simulink model "different_inverter_controls_BPS"  (R2024b)
settings: Solver=ode4  StartTime=0.0  StopTime=5  FixedStep=Ts  RelTol=1e-3
InitFcn:
  | %mode_of_operation=1;
  | %BESS_control_mode=1;
  | %Gen_Q_Control =1;
  | 
  | %Exciter_init;
  | 
  | %Exciter_init
  | Xq=0.474;
  | %%====================================================
  | % ST6C Exciter Parameters
  | 
  | KPA=30;
  | KIA=59.91;
  | KFF=1;
  | KM=1;
  | KLR=22.47;
  | KCL=1.04;
  | VAMAX=7.05;
  | VAMIN=-6.11;
  | VRMAX=7.05;
  | VRMIN=-6.11;
  | ILR=5.02;
  | KG=1;
  | TG=0.024;
  | TA=0.01;
  | VBMAX=999;
  | VMMAX=7.05;
  | VMMIN=-6.11;
  | KI=0;
  | Kp=1;
  | Kc=0;
  | Vt0=0;
  | VAAMAX=VAMAX;
  | %%========================================================
  | % UEL2C parameters
  | 
  | TUQ=.005;
  | TUP=0.050;
  | TUV=0.2;
  | TQREF=0;
  | Tadj=0;
  | K1=0;
  | K2=2;
  | VBIAS=1;
  | KFB=0;
  | TUL=0;
  | VUImax=1;
  | VUImin=-1;
  | VUELmax1=1;
  | VUELmax2=1;
  | VUELmin1=-1;
  | VUELmin2=-1;
  | KUF=0;
  | KUL=0.24;
  | KUI=0.001;
  | TU1=0;TU2=0;TU3=0;TU4=0;
  | KFIX=1;
  | VF=0;
  | VFB=0;
  | %%===========================================================
  | ... (+60 lines)
values from neighbouring files (symbols this model uses):
  inv1 = struct    [multiInverterParams.m]
  kp_sync = KQ_p/10    (= 0.04)    [multiInverterParams.m]
  Vdc = 1000    [multiInverterParams.m]
  Vpp = 480    [multiInverterParams.m]
undefined symbols (not defined in the file or in its folder): D1, Delta, DiscIntNeverNeededParam, Ion, Lithium, sigbuilder_block, sps
libraries: slpidlib x34, spsThreePhaseVIMeasurementLib x31, spsThreePhaseSeriesRLCBranchLib x23, spsabctodq0Lib x22, spsPower3phInstantaneousLib x22, spsThreePhaseTransformerTwoWindingsLib x16, spsSeriesRLCBranchLib x16, spsThreePhaseSeriesRLCLoadLib x14, simulink x12, spsPLL3phLib x11, spsGroundLib x9, powerlib_extras x8
(part 7 of 9)

== system different_inverter_controls_BPS/GFM-VSG-100MW/IBR-GFM VSG/Inverter/Power Controller/P,Q Control  ==
  PQref : Inport
  m : Inport  Port=2
  V_inv_mag : Inport  Port=3
  Constant2 : Constant  Value=0  SampleTime=Ts_Control
  Demux : Demux  Outputs=2
  Demux1 : Demux  Outputs=2
  Gain1 : Gain  Gain=77*10
  Integrator : Subsystem
  Reactive Controller : slpidlib/PID Controller  Controller=PI  Form=Parallel  TimeDomain=Discrete-time  UseExternalTs=off  SampleTime=Ts_Control  IntegratorMethod=Forward Euler  FilterMethod=Forward Euler  ControllerParametersSource=internal  P=-.001  I=0  UseKiTs=off  D=0  UseExternalDerivativeSource=off  N=100  UseFilter=on  TunerSelectOption=Transfer Function Based (PID Tuner App)  InitialConditionSource=internal  InitialConditionForIntegrator=0  InitialConditionForFilter=0  DifferentiatorICPrevScaledInput=0  ExternalReset=none  TrackingMode=off  Kt=1  LimitOutput=on  SatLimitsSource=internal  UpperSaturationLimit=1.5  LowerSaturationLimit=-1.5  LinearizeAsGain=off  AntiWindupMode=back-calculation  Kb=1  LimitIntegrator=off  UpperIntegratorSaturationLimit=inf  LowerIntegratorSaturationLimit=-inf  POutMin=[]  POutMax=[]  IOutMin=[]  IOutMax=[]  DOutMin=[]  DOutMax=[]  NOutMin=[]  NOutMax=[]  SumOutMin=[]  SumOutMax=[]  SaturationOutMin=[]  SaturationOutMax=[]  PParamMin=[]  PParamMax=[]  IParamMin=[]  IParamMax=[]  DParamMin=[]  DParamMax=[]  NParamMin=[]  NParamMax=[]  KbParamMin=[]  KbParamMax=[]  KtParamMin=[]  KtParamMax=[]  KbOutMin=[]  KbOutMax=[]  KtOutMin=[]  KtOutMax=[]  IntegratorOutMin=[]  IntegratorOutMax=[]  FilterOutMin=[]  FilterOutMax=[]  SumI1OutMin=[]  SumI1OutMax=[]  SumI2OutMin=[]  SumI2OutMax=[]  SumI3OutMin=[]  SumI3OutMax=[]  SumI4OutMin=[]  SumI4OutMax=[]  SumDOutMin=[]  SumDOutMax=[]  DifferentiatorOutMin=[]  DifferentiatorOutMax=[]  FilterDiffOutCoefMin=[]  FilterDiffOutCoefMax=[]  ReciprocalOutMin=[]  ReciprocalOutMax=[]  SumDenOutMin=[]  SumDenOutMax=[]  SumNumOutMin=[]  SumNumOutMax=[]  DivideOutMin=[]  DivideOutMax=[]  UdiffTsProdOutMin=[]  UdiffTsProdOutMax=[]  NTsProdOutMin=[]  NTsProdOutMax=[]  UintegralTsProdOutMin=[]  UintegralTsProdOutMax=[]  UngainTsProdOutMin=[]  UngainTsProdOutMax=[]  ClampingZeroOutDataTypeStr=Inherit: Inherit via back propagation  ClampingZeroOutMin=[]  ClampingZeroOutMax=[]  FilterDenConstantOutDataTypeStr=Inherit: Inherit via back propagation  FilterDenConstantOutMin=[]  FilterDenConstantOutMax=[]  PCopyOutDataTypeStr=Inherit: Inherit via back propagation  PCopyOutMin=[]  PCopyOutMax=[]  NCopyOutDataTypeStr=Inherit: Inherit via back propagation  NCopyOutMin=[]  NCopyOutMax=[]  IntegratorContinuousStateAttributes=''  IntegratorStateMustResolveToSignalObject=off  IntegratorRTWStateStorageClass=Auto  FilterContinuousStateAttributes=''  FilterStateMustResolveToSignalObject=off  FilterRTWStateStorageClass=Auto  ParallelPVariant=InternalParameters  IdealPVariant=Disabled  IVariant=InternalParameters  DVariant=Disabled  IntegratorVariant=Discrete  SatVariant=Enabled  AWVariant=BackCalculation  PCopyVariant=Disabled  TRVariant=Disabled  FdbkBlocksVariant=Forward  IdealPFdbkVariant=Disabled  SatFdbkVariant=Disabled  DerivativeFilterVariant=Disabled  NVariant=Disabled  NCopyVariant=Disabled_SignalSpec  FilterICVariant=Disabled  IntegratorICVariant=InternalICs  ExternalResetVariant=Disabled  TRSumVariant=Passthrough  SumFdbkVariant=Disabled  SumVariant=Sum_PI  TsampFilterVariant=InternalTs  TsampNgainVariant=Passthrough  TsampIntegralVariant=Disabled_SignalSpec  ExternalSaturationOutDataTypeStr=Inherit: Same as second input  DerivativeSourceVariant=Disabled  PreIntVariant=InternalPreInt
  Scope{1,3,6..9} (6 alike) : Scope
  Scope10 : Scope  NumInputPorts=2
  Scope2 : Scope  NumInputPorts=2
  Sum : Sum  Inputs=|+-
  Sum1 : Sum  Inputs=|+-
  Sum2 : Sum  Inputs=-+
  Sum3 : Sum  Inputs=|++
  Sum5 : Sum  Inputs=|+-
  Transfer Fcn3 : TransferFcn  Denominator=[15 0]
  V0 : Constant  SampleTime=Ts_Control
  passing flag2 : Switch  Threshold=0.9  SaturateOnIntegerOverflow=off  InputSameDT=off
  w01 : Constant  SampleTime=Ts_Control
  theta : Outport  VectorParamsAs1DForOutWhenUnconnected=off
  Vdref : Outport  Port=2
  wires:
  Integrator/1(Theta) -> Scope3/1, theta/1
  Demux1/1 -> Sum/2, Scope8/1
  m/1 -> Demux1/1
  PQref/1 -> Demux/1
  Demux/1 -> Scope7/1, Sum/1  "Pref"
  Demux/2 -> Sum2/1, Scope6/1  "Qref"
  Demux1/2 -> Sum2/2, Scope1/1
  Sum2/1 -> Scope10/1, Reactive Controller/1
  Reactive Controller/1 -> Scope10/2, Sum3/1
  V0/1 -> Sum3/2
  Sum3/1 -> Scope9/1, Vdref/1  "vdref"
  V_inv_mag/1 -> passing flag2/2
  Constant2/1 -> passing flag2/3
  Sum5/1 -> Gain1/1
  Gain1/1 -> Sum1/2
  Sum1/1 -> Transfer Fcn3/1
  Transfer Fcn3/1 -> Integrator/1(w), Scope2/2, Sum5/1
  Sum/1 -> passing flag2/1
  passing flag2/1 -> Sum1/1, Scope2/1
  w01/1 -> Sum5/2

== system different_inverter_controls_BPS/GT-swing/Gen-a/Synchronous Machine G2 50 MVA 16.5 kV/Governor model with Droop/gen outage ==
  Input : Inport
  Product : Product
  Step : Step  Time=50  Before=1  After=0  SampleTime=Ts
  Output : Outport
  wires:
  Product/1 -> Output/1
  Input/1 -> Product/1
  Step/1 -> Product/2

== system different_inverter_controls_BPS/IBR GFL-SH/BESS/Inverter Control/Current Control/Current Regulator ==
  note: Id positive --> The converter generates active power ("Inverter mode") = Active Power P positive
  note: Iq positive --> The converter absorbs reactive power ("Inductive mode") = Reactive Power Q negative
  note: Sign Convention: Current going out of the converter = positive current
  note: Current Regulator
      | ================
  VdVq_meas : Inport  PortDimensions=2
  IdIq_meas : Inport  Port=2  PortDimensions=2
  IdIq_ref : Inport  Port=3  PortDimensions=2
  Add1 : Sum  Inputs=++-
  Add2 : Sum
  Add3 : Sum  Inputs=+++
  Demux : Demux  Outputs=2
  Demux1 : Demux  Outputs=2
  Lff : Gain  Gain=Ltot_pu  SaturateOnIntegerOverflow=on  OutDataTypeStr=Inherit: Same as input  ParamDataTypeStr=Inherit: Same as input
  "Lff  " : Gain  Gain=Ltot_pu  SaturateOnIntegerOverflow=on  OutDataTypeStr=Inherit: Same as input  ParamDataTypeStr=Inherit: Same as input
  Mux : Mux  Inputs=2
  PI : slpidlib/PID Controller  Controller=PI  Form=Parallel  TimeDomain=Discrete-time  UseExternalTs=off  SampleTime=Ts_Control  IntegratorMethod=Forward Euler  FilterMethod=Forward Euler  ControllerParametersSource=internal  P=Kp_Ireg  I=Ki_Ireg  D=0  UseFilter=on  N=100  TunerSelectOption=Transfer Function Based (PID Tuner App)  InitialConditionSource=internal  InitialConditionForIntegrator=0  InitialConditionForFilter=0  DifferentiatorICPrevScaledInput=0  ExternalReset=none  TrackingMode=off  Kt=1  LimitOutput=on  SatLimitsSource=internal  UpperSaturationLimit=1.5  LowerSaturationLimit=-1.5  LinearizeAsGain=off  AntiWindupMode=clamping  Kb=1  POutMin=[]  POutMax=[]  IOutMin=[]  IOutMax=[]  DOutMin=[]  DOutMax=[]  NOutMin=[]  NOutMax=[]  SumOutMin=[]  SumOutMax=[]  SaturationOutMin=[]  SaturationOutMax=[]  PParamMin=[]  PParamMax=[]  IParamMin=[]  IParamMax=[]  DParamMin=[]  DParamMax=[]  NParamMin=[]  NParamMax=[]  KbParamMin=[]  KbParamMax=[]  KtParamMin=[]  KtParamMax=[]  KbOutMin=[]  KbOutMax=[]  KtOutMin=[]  KtOutMax=[]  IntegratorOutMin=[]  IntegratorOutMax=[]  FilterOutMin=[]  FilterOutMax=[]  SumI1OutMin=[]  SumI1OutMax=[]  SumI2OutMin=[]  SumI2OutMax=[]  SumI3OutMin=[]  SumI3OutMax=[]  SumI4OutMin=[]  SumI4OutMax=[]  SumDOutMin=[]  SumDOutMax=[]  DifferentiatorOutMin=[]  DifferentiatorOutMax=[]  FilterDiffOutCoefMin=[]  FilterDiffOutCoefMax=[]  ReciprocalOutMin=[]  ReciprocalOutMax=[]  SumDenOutMin=[]  SumDenOutMax=[]  SumNumOutMin=[]  SumNumOutMax=[]  DivideOutMin=[]  DivideOutMax=[]  UdiffTsProdOutMin=[]  UdiffTsProdOutMax=[]  NTsProdOutMin=[]  NTsProdOutMax=[]  UintegralTsProdOutMin=[]  UintegralTsProdOutMax=[]  UngainTsProdOutMin=[]  UngainTsProdOutMax=[]  IntegratorContinuousStateAttributes=''  IntegratorStateMustResolveToSignalObject=off  IntegratorRTWStateStorageClass=Auto  FilterContinuousStateAttributes=''  FilterStateMustResolveToSignalObject=off  FilterRTWStateStorageClass=Auto  ParallelPVariant=InternalParameters  IdealPVariant=Disabled  IVariant=InternalParameters  DVariant=Disabled  IntegratorVariant=Discrete  SatVariant=Enabled  AWVariant=DiscClampingParallel  PCopyVariant=Disabled  TRVariant=Disabled  FdbkBlocksVariant=Forward  IdealPFdbkVariant=Disabled  SatFdbkVariant=Disabled  DerivativeFilterVariant=Disabled  NVariant=Disabled  NCopyVariant=Disabled_SignalSpec  FilterICVariant=Disabled  IntegratorICVariant=InternalICs  ExternalResetVariant=Disabled  TRSumVariant=Passthrough  SumFdbkVariant=Disabled  SumVariant=Sum_PI  TsampFilterVariant=InternalTs  TsampNgainVariant=Passthrough  TsampIntegralVariant=Passthrough  ExternalSaturationOutDataTypeStr=Inherit: Same as second input
  Rff : Gain  Gain=Rtot_pu  SaturateOnIntegerOverflow=on  OutDataTypeStr=Inherit: Same as input  ParamDataTypeStr=Inherit: Same as input
  "Rff " : Gain  Gain=Rtot_pu  SaturateOnIntegerOverflow=on  OutDataTypeStr=Inherit: Same as input  ParamDataTypeStr=Inherit: Same as input
  Saturation : Saturate  UpperLimit=1.5  LowerLimit=-1.5
  Scope : Scope  NumInputPorts=2
  Sum : Sum  Inputs=|-+
  VdVq_conv : Outport  VectorParamsAs1DForOutWhenUnconnected=off
  wires:
  Add3/1 -> Mux/2
  Demux/2 -> Add3/1
  Add1/1 -> Mux/1  "Feedforward"
  Lff/1 -> Add3/3
  Rff/1 -> Add3/2
  Demux1/2 -> Rff/1, "Lff  "/1
  "Lff  "/1 -> Add1/3
  Demux1/1 -> Lff/1, "Rff "/1
  "Rff "/1 -> Add1/2
  Demux/1 -> Add1/1
  VdVq_meas/1 -> Demux/1
  Saturation/1 -> VdVq_conv/1
  Add2/1 -> Saturation/1
  IdIq_meas/1 -> Sum/1
  IdIq_ref/1 -> Demux1/1, Sum/2
  Sum/1 -> PI/1, Scope/1
  PI/1 -> Add2/1, Scope/2  "PI"
  Mux/1 -> Add2/2

== system different_inverter_controls_BPS/IBR GFL-SH/BESS/Inverter Control/Current Control/Uabc_ref Generation max (m) = 1 ==
  note: Uref Generation
      | ==============
  note: (Correction for delai of Ts_Control)
  note: (Correction for transformer
      |  D1 connection)
  wt : Inport
  VdVq_conv : Inport  Port=2
  Add1 : Sum  Inputs=++++
  Add2 : Sum
  Complex to Magnitude-Angle : ComplexToMagnitudeAngle
  Constant : Constant  Value=-pi/6
  Constant1 : Constant  Value=Vnom_dc
  Constant2 : Constant  Value="[ 0  -2*pi/3  2*pi/3  ]"
  Constant3 : Constant  Value=Vnom_sec*sqrt(2)/sqrt(3)
  Constant4 : Constant  Value=Ts_Control*Fnom*(2*pi)
  Demux1 : Demux  Outputs=2
  Gain1 : Gain  Gain=1/2
  Product : Product  Inputs=*/  RndMeth=Zero
  Product1 : Product  Inputs=*/  RndMeth=Zero
  Product2 : Product  Inputs=**  RndMeth=Zero
  Real-Imag to Complex : RealImagToComplex
  Trigonometric Function : Trigonometry
  Uabc_ref : Outport  VectorParamsAs1DForOutWhenUnconnected=off
  wires:
  Constant4/1 -> Add1/4
  wt/1 -> Add1/1
  Product2/1 -> Uabc_ref/1
  Trigonometric Function/1 -> Product2/2
  Complex to Magnitude-Angle/1 -> Product2/1
  Add2/1 -> Trigonometric Function/1
  Add1/1 -> Add2/2
  Complex to Magnitude-Angle/2 -> Add2/1
  Product/1 -> Product1/2
  Constant3/1 -> Product/2
  Constant/1 -> Add1/3
  Constant2/1 -> Add1/2
  Demux1/2 -> Real-Imag to Complex/2
  Demux1/1 -> Real-Imag to Complex/1
  Real-Imag to Complex/1 -> Complex to Magnitude-Angle/1
  Gain1/1 -> Product/1
  Product1/1 -> Demux1/1
  VdVq_conv/1 -> Product1/1
  Constant1/1 -> Gain1/1

== system different_inverter_controls_BPS/IBR GFL-SH/BESS/Inverter Control/current limiter/P priority limit ==
  idiqP : Inport
  Demux4 : Demux  Outputs=2
  IqLimit : Subsystem
  Mux4 : Mux  Inputs=2
  Rtot_pu1 : Gain  Gain=-1  SaturateOnIntegerOverflow=on  OutDataTypeStr=Inherit: Same as input  ParamDataTypeStr=Inherit: Same as input
  Saturation : Saturate  UpperLimit=limMax  LowerLimit=0
  Saturation Dynamic : simulink/Discontinuities/Saturation Dynamic  OutMin=[]  OutMax=[]  OutDataTypeStr=Inherit: Same as second input  OutDataType=fixdt(1, 16)  OutScaling=2^-10  DoSatur=off
  Out1 : Outport
  wires:
  IqLimit/1(Out2) -> Saturation Dynamic/1, Rtot_pu1/1
  Rtot_pu1/1 -> Saturation Dynamic/3
  Saturation/1 -> Mux4/1, IqLimit/1(In1)
  Demux4/1 -> Saturation/1
  Mux4/1 -> Out1/1
  Demux4/2 -> Saturation Dynamic/2
  idiqP/1 -> Demux4/1
  Saturation Dynamic/1 -> Mux4/2

== system different_inverter_controls_BPS/IBR GFL-SH/BESS/Inverter Control/current limiter/Q priority limit ==
  idiqP : Inport
  Demux4 : Demux  Outputs=2
  IqLimit : Subsystem
  Mux4 : Mux  Inputs=2
  Rtot_pu1 : Gain  Gain=-1  SaturateOnIntegerOverflow=on  OutDataTypeStr=Inherit: Same as input  ParamDataTypeStr=Inherit: Same as input
  Saturation : Saturate  UpperLimit=limMax  LowerLimit=0
  Saturation Dynamic : simulink/Discontinuities/Saturation Dynamic  OutMin=[]  OutMax=[]  OutDataTypeStr=Inherit: Same as second input  OutDataType=fixdt(1, 16)  OutScaling=2^-10  DoSatur=off
  Out1 : Outport
  wires:
  Saturation/1 -> IqLimit/1(In1), Mux4/2
  Demux4/2 -> Saturation/1
  Demux4/1 -> Saturation Dynamic/2
  Saturation Dynamic/1 -> Mux4/1
  IqLimit/1(Out2) -> Saturation Dynamic/1, Rtot_pu1/1
  Rtot_pu1/1 -> Saturation Dynamic/3
  Mux4/1 -> Out1/1
  idiqP/1 -> Demux4/1

== system different_inverter_controls_BPS/IBR GFL-SH/BESS/Inverter Control/current limiter/Subsystem3 ==
  In1 : Inport
  Demux2 : Demux  Outputs=2
  Math Function : Math  Operator=square  SignedPower=on
  Saturation : Saturate  UpperLimit=limMax  LowerLimit=limMin
  Scope : Scope  NumInputPorts=2
  Sqrt1 : Sqrt
  Subtract : Sum
  Out1 : Outport
  Out2 : Outport  Port=2
  wires:
  Saturation/1 -> Out1/1
  Sqrt1/1 -> Out2/1, Scope/1, Saturation/1
  Subtract/1 -> Sqrt1/1  "Ipos2"
  In1/1 -> Math Function/1, Scope/2
  Math Function/1 -> Demux2/1
  Demux2/1 -> Subtract/1
  Demux2/2 -> Subtract/2

== system different_inverter_controls_BPS/IBR GFL-SH/BESS/Inverter Control/current limiter/Subsystem4 ==
  In1 : Inport
  In2 : Inport  Port=2
  Demux4 : Demux  Outputs=2
  Mux4 : Mux  Inputs=2
  Switch1 : Switch  Threshold=limMax  SaturateOnIntegerOverflow=off  InputSameDT=off
  Unit Delay2 : UnitDelay  InitialCondition=1  SampleTime=Ts_Control  HasFrameUpgradeWarning=on
  dummy limit : Saturate  UpperLimit=limMax  LowerLimit=limMin
  Out1 : Outport
  wires:
  dummy limit/1 -> Mux4/2
  Demux4/2 -> dummy limit/1
  In2/1 -> Demux4/1, Switch1/3
  In1/1 -> Switch1/2
  Unit Delay2/1 -> Switch1/1
  Switch1/1 -> Unit Delay2/1, Mux4/1, Out1/1

== system different_inverter_controls_BPS/IBR GFL-SH/BESS/Inverter Control/current limiter/Subsystem9 ==
  In1 : Inport
  In2 : Inport  Port=2
  Divide : Product  Inputs=*/
  Gain1 : Gain  Gain=limMax
  Saturation : Saturate  UpperLimit=limMax  LowerLimit=limMin
  Switch1 : Switch  Threshold=limMax  SaturateOnIntegerOverflow=off  InputSameDT=off
  Out1 : Outport
  wires:
  Saturation/1 -> Out1/1
  Switch1/1 -> Saturation/1
  Gain1/1 -> Switch1/1
  Divide/1 -> Gain1/1
  In2/1 -> Switch1/3, Divide/1
  In1/1 -> Switch1/2, Divide/2

== system different_inverter_controls_BPS/IBR GFL-SH/IBR/ Reference /Pref/Signal Builder ==
  Demux : Demux  Tag=STV Demux  Outputs=2
      settings: DisplayOption=none
  FromWs : FromWorkspace  Tag=STV FromWs  VariableName=tuvar
      SigBuilderData=|
      | common.afterFinalStr = 'Extrapolate'
      | common.sampleTime = 0
      | dataSet.timeRange = [0 24]
      | dataSet.name = 'Group 1'
      | sbobj.Groups.Name = 'Group 1'
      | sbobj.Groups.Signals(1).Name = 'Signal 2'
      | sbobj.Groups.Signals(1).XData = [0 3 3 6 6 9 11.35 11.35 20 24]
      | sbobj.Groups.Signals(1).YData = [40 40 0.5 0.5 0 23.5 23.5 40 41 41]
      | sbobj.Groups.Signals(2).Name = 'Signal 1'
      | sbobj.Groups.Signals(2).XData = [0 1 2 3 4 5 6 7 8 9 10 11 12 13 14 15 16 17 18 19 24]
      | sbobj.Groups.Signals(2).YData = [0 0 0 0 0 0 0.1 0.2 0.3 0.5 0.8 0.9 1 1 0.99 0.9 0.7 0.4 0.1 0 0]
      | sbobj.Groups.TimeRange = [0 24]
  Signal 2 : Outport  Tag=STV Outport
  Signal 1 : Outport  Tag=STV Outport  Port=2
  wires:
  FromWs/1 -> Demux/1
  Demux/1 -> Signal 2/1
  Demux/2 -> Signal 1/1

== system different_inverter_controls_BPS/IBR GFL-SH/IBR/ Reference /Qref/Signal Builder ==
  Demux : Demux  Tag=STV Demux  Outputs=1
      settings: DisplayOption=none
  FromWs : FromWorkspace  Tag=STV FromWs  VariableName=tuvar
      SigBuilderData=|
      | common.afterFinalStr = 'Extrapolate'
      | common.sampleTime = 0
      | dataSet.timeRange = [0 20]
      | dataSet.name = 'Group 1'
      | sbobj.Groups.Name = 'Group 1'
      | sbobj.Groups.Signals.Name = 'Signal 2'
      | sbobj.Groups.Signals.XData = [0 3 3 6 6 9 9 12 12 20]
      | sbobj.Groups.Signals.YData = [10 10 -10 -10 15 15 40 40 10 10.2]
      | sbobj.Groups.TimeRange = [0 20]
  Signal 2 : Outport  Tag=STV Outport
  wires:
  FromWs/1 -> Demux/1
  Demux/1 -> Signal 2/1

== system different_inverter_controls_BPS/IBR GFL-SH/IBR/Inverter Control/Current Control/Current Regulator ==
  note: Id positive --> The converter generates active power ("Inverter mode") = Active Power P positive
  note: Iq positive --> The converter absorbs reactive power ("Inductive mode") = Reactive Power Q negative
  note: Sign Convention: Current going out of the converter = positive current
  note: Current Regulator
      | ================
  VdVq_meas : Inport  PortDimensions=2
  IdIq_meas : Inport  Port=2  PortDimensions=2
  IdIq_ref : Inport  Port=3  PortDimensions=2
  Add1 : Sum  Inputs=++-
  Add2 : Sum
  Add3 : Sum  Inputs=+++
  Demux : Demux  Outputs=2
  Demux1 : Demux  Outputs=2
  Lff : Gain  Gain=Ltot_pu  SaturateOnIntegerOverflow=on  OutDataTypeStr=Inherit: Same as input  ParamDataTypeStr=Inherit: Same as input
  "Lff  " : Gain  Gain=Ltot_pu  SaturateOnIntegerOverflow=on  OutDataTypeStr=Inherit: Same as input  ParamDataTypeStr=Inherit: Same as input
  Mux : Mux  Inputs=2
  PI : slpidlib/PID Controller  Controller=PI  Form=Parallel  TimeDomain=Discrete-time  UseExternalTs=off  SampleTime=Ts_Control  IntegratorMethod=Forward Euler  FilterMethod=Forward Euler  ControllerParametersSource=internal  P=Kp_Ireg  I=Ki_Ireg  D=0  UseFilter=on  N=100  TunerSelectOption=Transfer Function Based (PID Tuner App)  InitialConditionSource=internal  InitialConditionForIntegrator=0  InitialConditionForFilter=0  DifferentiatorICPrevScaledInput=0  ExternalReset=none  TrackingMode=off  Kt=1  LimitOutput=on  SatLimitsSource=internal  UpperSaturationLimit=1.5  LowerSaturationLimit=-1.5  LinearizeAsGain=off  AntiWindupMode=clamping  Kb=1  POutMin=[]  POutMax=[]  IOutMin=[]  IOutMax=[]  DOutMin=[]  DOutMax=[]  NOutMin=[]  NOutMax=[]  SumOutMin=[]  SumOutMax=[]  SaturationOutMin=[]  SaturationOutMax=[]  PParamMin=[]  PParamMax=[]  IParamMin=[]  IParamMax=[]  DParamMin=[]  DParamMax=[]  NParamMin=[]  NParamMax=[]  KbParamMin=[]  KbParamMax=[]  KtParamMin=[]  KtParamMax=[]  KbOutMin=[]  KbOutMax=[]  KtOutMin=[]  KtOutMax=[]  IntegratorOutMin=[]  IntegratorOutMax=[]  FilterOutMin=[]  FilterOutMax=[]  SumI1OutMin=[]  SumI1OutMax=[]  SumI2OutMin=[]  SumI2OutMax=[]  SumI3OutMin=[]  SumI3OutMax=[]  SumI4OutMin=[]  SumI4OutMax=[]  SumDOutMin=[]  SumDOutMax=[]  DifferentiatorOutMin=[]  DifferentiatorOutMax=[]  FilterDiffOutCoefMin=[]  FilterDiffOutCoefMax=[]  ReciprocalOutMin=[]  ReciprocalOutMax=[]  SumDenOutMin=[]  SumDenOutMax=[]  SumNumOutMin=[]  SumNumOutMax=[]  DivideOutMin=[]  DivideOutMax=[]  UdiffTsProdOutMin=[]  UdiffTsProdOutMax=[]  NTsProdOutMin=[]  NTsProdOutMax=[]  UintegralTsProdOutMin=[]  UintegralTsProdOutMax=[]  UngainTsProdOutMin=[]  UngainTsProdOutMax=[]  FilterDenConstantOutDataTypeStr=Inherit: Inherit via back propagation  FilterDenConstantOutMin=[]  FilterDenConstantOutMax=[]  PCopyOutDataTypeStr=Inherit: Inherit via back propagation  PCopyOutMin=[]  PCopyOutMax=[]  NCopyOutDataTypeStr=Inherit: Inherit via back propagation  NCopyOutMin=[]  NCopyOutMax=[]  IntegratorContinuousStateAttributes=''  IntegratorStateMustResolveToSignalObject=off  IntegratorRTWStateStorageClass=Auto  FilterContinuousStateAttributes=''  FilterStateMustResolveToSignalObject=off  FilterRTWStateStorageClass=Auto  ParallelPVariant=InternalParameters  IdealPVariant=Disabled  IVariant=InternalParameters  DVariant=Disabled  IntegratorVariant=Discrete  SatVariant=Enabled  AWVariant=DiscClampingParallel  PCopyVariant=Disabled  TRVariant=Disabled  FdbkBlocksVariant=Forward  IdealPFdbkVariant=Disabled  SatFdbkVariant=Disabled  DerivativeFilterVariant=Disabled  NVariant=Disabled  NCopyVariant=Disabled_SignalSpec  FilterICVariant=Disabled  IntegratorICVariant=InternalICs  ExternalResetVariant=Disabled  TRSumVariant=Passthrough  SumFdbkVariant=Disabled  SumVariant=Sum_PI  TsampFilterVariant=InternalTs  TsampNgainVariant=Passthrough  TsampIntegralVariant=Passthrough  ExternalSaturationOutDataTypeStr=Inherit: Same as second input
  Rff : Gain  Gain=Rtot_pu  SaturateOnIntegerOverflow=on  OutDataTypeStr=Inherit: Same as input  ParamDataTypeStr=Inherit: Same as input
  "Rff " : Gain  Gain=Rtot_pu  SaturateOnIntegerOverflow=on  OutDataTypeStr=Inherit: Same as input  ParamDataTypeStr=Inherit: Same as input
  Saturation : Saturate  UpperLimit=1.5  LowerLimit=-1.5
  Scope : Scope  NumInputPorts=2
  Sum : Sum  Inputs=|-+
  VdVq_conv : Outport  VectorParamsAs1DForOutWhenUnconnected=off
  wires:
  Add3/1 -> Mux/2
  Demux/2 -> Add3/1
  Add1/1 -> Mux/1  "Feedforward"
  Lff/1 -> Add3/3
  Rff/1 -> Add3/2
  Demux1/2 -> Rff/1, "Lff  "/1
  "Lff  "/1 -> Add1/3
  Demux1/1 -> Lff/1, "Rff "/1
  "Rff "/1 -> Add1/2
  Demux/1 -> Add1/1
  VdVq_meas/1 -> Demux/1
  Saturation/1 -> VdVq_conv/1
  Add2/1 -> Saturation/1
  IdIq_meas/1 -> Sum/1
  IdIq_ref/1 -> Demux1/1, Sum/2
  Sum/1 -> PI/1, Scope/1
  PI/1 -> Add2/1, Scope/2  "PI"
  Mux/1 -> Add2/2

== system different_inverter_controls_BPS/IBR GFL-SH/IBR/Inverter Control/Current Control/Uabc_ref Generation max (m) = 1 ==
  note: Uref Generation
      | ==============
  note: (Correction for delai of Ts_Control)
  note: (Correction for transformer
      |  D1 connection)
  wt : Inport
  VdVq_conv : Inport  Port=2
  Add1 : Sum  Inputs=++++
  Add2 : Sum
  Complex to Magnitude-Angle : ComplexToMagnitudeAngle
  Constant : Constant  Value=-pi/6
  Constant1 : Constant  Value=Vnom_dc
  Constant2 : Constant  Value="[ 0  -2*pi/3  2*pi/3  ]"
  Constant3 : Constant  Value=Vnom_sec*sqrt(2)/sqrt(3)
  Constant4 : Constant  Value=Ts_Control*Fnom*(2*pi)
  Demux1 : Demux  Outputs=2
  Gain1 : Gain  Gain=1/2
  Product : Product  Inputs=*/  RndMeth=Zero
  Product1 : Product  Inputs=*/  RndMeth=Zero
  Product2 : Product  Inputs=**  RndMeth=Zero
  Real-Imag to Complex : RealImagToComplex
  Trigonometric Function : Trigonometry
  Uabc_ref : Outport  VectorParamsAs1DForOutWhenUnconnected=off
  wires:
  Constant4/1 -> Add1/4
  wt/1 -> Add1/1
  Product2/1 -> Uabc_ref/1
  Trigonometric Function/1 -> Product2/2
  Complex to Magnitude-Angle/1 -> Product2/1
  Add2/1 -> Trigonometric Function/1
  Add1/1 -> Add2/2
  Complex to Magnitude-Angle/2 -> Add2/1
  Product/1 -> Product1/2
  Constant3/1 -> Product/2
  Constant/1 -> Add1/3
  Constant2/1 -> Add1/2
  Demux1/2 -> Real-Imag to Complex/2
  Demux1/1 -> Real-Imag to Complex/1
  Real-Imag to Complex/1 -> Complex to Magnitude-Angle/1
  Gain1/1 -> Product/1
  Product1/1 -> Demux1/1
  VdVq_conv/1 -> Product1/1
  Constant1/1 -> Gain1/1

== system different_inverter_controls_BPS/IBR GFL-SH/IBR/Inverter Control/current limiter/P priority limit ==
  idiqP : Inport
  Demux4 : Demux  Outputs=2
  IqLimit : Subsystem
  Mux4 : Mux  Inputs=2
  Rtot_pu1 : Gain  Gain=-1  SaturateOnIntegerOverflow=on  OutDataTypeStr=Inherit: Same as input  ParamDataTypeStr=Inherit: Same as input
  Saturation : Saturate  UpperLimit=limMax  LowerLimit=0
  Saturation Dynamic : simulink/Discontinuities/Saturation Dynamic  OutMin=[]  OutMax=[]  OutDataTypeStr=Inherit: Same as second input  OutDataType=fixdt(1, 16)  OutScaling=2^-10  DoSatur=off
  Out1 : Outport
  wires:
  IqLimit/1(Out2) -> Saturation Dynamic/1, Rtot_pu1/1
  Rtot_pu1/1 -> Saturation Dynamic/3
  Saturation/1 -> Mux4/1, IqLimit/1(In1)
  Demux4/1 -> Saturation/1
  Mux4/1 -> Out1/1
  Demux4/2 -> Saturation Dynamic/2
  idiqP/1 -> Demux4/1
  Saturation Dynamic/1 -> Mux4/2

== system different_inverter_controls_BPS/IBR GFL-SH/IBR/Inverter Control/current limiter/Q priority limit ==
  idiqP : Inport
  Demux4 : Demux  Outputs=2
  IqLimit : Subsystem
  Mux4 : Mux  Inputs=2
  Rtot_pu1 : Gain  Gain=-1  SaturateOnIntegerOverflow=on  OutDataTypeStr=Inherit: Same as input  ParamDataTypeStr=Inherit: Same as input
  Saturation : Saturate  UpperLimit=limMax  LowerLimit=0
  Saturation Dynamic : simulink/Discontinuities/Saturation Dynamic  OutMin=[]  OutMax=[]  OutDataTypeStr=Inherit: Same as second input  OutDataType=fixdt(1, 16)  OutScaling=2^-10  DoSatur=off
  Out1 : Outport
  wires:
  Saturation/1 -> IqLimit/1(In1), Mux4/2
  Demux4/2 -> Saturation/1
  Demux4/1 -> Saturation Dynamic/2
  Saturation Dynamic/1 -> Mux4/1
  IqLimit/1(Out2) -> Saturation Dynamic/1, Rtot_pu1/1
  Rtot_pu1/1 -> Saturation Dynamic/3
  Mux4/1 -> Out1/1
  idiqP/1 -> Demux4/1

== system different_inverter_controls_BPS/IBR GFL-SH/IBR/Inverter Control/current limiter/Subsystem3 ==
  In1 : Inport
  Demux2 : Demux  Outputs=2
  Math Function : Math  Operator=square  SignedPower=on
  Saturation : Saturate  UpperLimit=limMax  LowerLimit=limMin
  Scope : Scope  NumInputPorts=2
  Sqrt1 : Sqrt
  Subtract : Sum
  Out1 : Outport
  Out2 : Outport  Port=2
  wires:
  Saturation/1 -> Out1/1
  Sqrt1/1 -> Out2/1, Scope/1, Saturation/1
  Subtract/1 -> Sqrt1/1  "Ipos2"
  In1/1 -> Math Function/1, Scope/2
  Math Function/1 -> Demux2/1
  Demux2/1 -> Subtract/1
  Demux2/2 -> Subtract/2

== system different_inverter_controls_BPS/IBR GFL-SH/IBR/Inverter Control/current limiter/Subsystem4 ==
  In1 : Inport
  In2 : Inport  Port=2
  Demux4 : Demux  Outputs=2
  Mux4 : Mux  Inputs=2
  Switch1 : Switch  Threshold=limMax  SaturateOnIntegerOverflow=off  InputSameDT=off
  Unit Delay2 : UnitDelay  InitialCondition=1  SampleTime=Ts_Control  HasFrameUpgradeWarning=on
  dummy limit : Saturate  UpperLimit=limMax  LowerLimit=limMin
  Out1 : Outport
  wires:
  dummy limit/1 -> Mux4/2
  Demux4/2 -> dummy limit/1
  In2/1 -> Demux4/1, Switch1/3
  In1/1 -> Switch1/2
  Unit Delay2/1 -> Switch1/1
  Switch1/1 -> Unit Delay2/1, Mux4/1, Out1/1

== system different_inverter_controls_BPS/IBR GFL-SH/IBR/Inverter Control/current limiter/Subsystem9 ==
  In1 : Inport
  In2 : Inport  Port=2
  Divide : Product  Inputs=*/
  Gain1 : Gain  Gain=limMax
  Saturation : Saturate  UpperLimit=limMax  LowerLimit=limMin
  Switch1 : Switch  Threshold=limMax  SaturateOnIntegerOverflow=off  InputSameDT=off
  Out1 : Outport
  wires:
  Saturation/1 -> Out1/1
  Switch1/1 -> Saturation/1
  Gain1/1 -> Switch1/1
  Divide/1 -> Gain1/1
  In2/1 -> Switch1/3, Divide/1
  In1/1 -> Switch1/2, Divide/2

== system different_inverter_controls_BPS/IBR-GFM PV Droop/IBR/Inverter Control/Current Control/Current Regulator ==
  note: Current Regulator
      | ================
  note: Sign Convention: Current going out of the converter = positive current
  note: Iq positive --> The converter absorbs reactive power ("Inductive mode") = Reactive Power Q negative
  note: Id positive --> The converter generates active power ("Inverter mode") = Active Power P positive
  VdVq_meas : Inport  PortDimensions=2
  IdIq_meas : Inport  Port=2  PortDimensions=2
  IdIq_ref : Inport  Port=3  PortDimensions=2
  Add1 : Sum  Inputs=++-
  Add2 : Sum
  Add3 : Sum  Inputs=+++
  Demux : Demux  Outputs=2
  Demux1 : Demux  Outputs=2
  Lff : Gain  Gain=inv1.Lpu  SaturateOnIntegerOverflow=on  OutDataTypeStr=Inherit: Same as input  ParamDataTypeStr=Inherit: Same as input
  "Lff  " : Gain  Gain=inv1.Lpu  SaturateOnIntegerOverflow=on  OutDataTypeStr=Inherit: Same as input  ParamDataTypeStr=Inherit: Same as input
  Lff  1 : Gain  Commented=on  Gain=Ltot_pu  SaturateOnIntegerOverflow=on  OutDataTypeStr=Inherit: Same as input  ParamDataTypeStr=Inherit: Same as input
  Mux : Mux  Inputs=2
  PI : slpidlib/PID Controller  Controller=PI  Form=Parallel  TimeDomain=Discrete-time  UseExternalTs=off  SampleTime=Ts_Control  IntegratorMethod=Forward Euler  FilterMethod=Forward Euler  ControllerParametersSource=internal  P=Kp_Ireg/10  I=Ki_Ireg  UseKiTs=off  D=0  UseExternalDerivativeSource=off  N=100  UseFilter=on  TunerSelectOption=Transfer Function Based (PID Tuner App)  InitialConditionSource=internal  InitialConditionForIntegrator=0  InitialConditionForFilter=0  DifferentiatorICPrevScaledInput=0  ExternalReset=none  TrackingMode=off  Kt=1  LimitOutput=on  SatLimitsSource=internal  UpperSaturationLimit=1.5  LowerSaturationLimit=-1.5  LinearizeAsGain=off  AntiWindupMode=back-calculation  Kb=1  LimitIntegrator=off  UpperIntegratorSaturationLimit=inf  LowerIntegratorSaturationLimit=-inf  POutMin=[]  POutMax=[]  IOutMin=[]  IOutMax=[]  DOutMin=[]  DOutMax=[]  NOutMin=[]  NOutMax=[]  SumOutMin=[]  SumOutMax=[]  SaturationOutMin=[]  SaturationOutMax=[]  PParamMin=[]  PParamMax=[]  IParamMin=[]  IParamMax=[]  DParamMin=[]  DParamMax=[]  NParamMin=[]  NParamMax=[]  KbParamMin=[]  KbParamMax=[]  KtParamMin=[]  KtParamMax=[]  KbOutMin=[]  KbOutMax=[]  KtOutMin=[]  KtOutMax=[]  IntegratorOutMin=[]  IntegratorOutMax=[]  FilterOutMin=[]  FilterOutMax=[]  SumI1OutMin=[]  SumI1OutMax=[]  SumI2OutMin=[]  SumI2OutMax=[]  SumI3OutMin=[]  SumI3OutMax=[]  SumI4OutMin=[]  SumI4OutMax=[]  SumDOutMin=[]  SumDOutMax=[]  DifferentiatorOutMin=[]  DifferentiatorOutMax=[]  FilterDiffOutCoefMin=[]  FilterDiffOutCoefMax=[]  ReciprocalOutMin=[]  ReciprocalOutMax=[]  SumDenOutMin=[]  SumDenOutMax=[]  SumNumOutMin=[]  SumNumOutMax=[]  DivideOutMin=[]  DivideOutMax=[]  UdiffTsProdOutMin=[]  UdiffTsProdOutMax=[]  NTsProdOutMin=[]  NTsProdOutMax=[]  UintegralTsProdOutMin=[]  UintegralTsProdOutMax=[]  UngainTsProdOutMin=[]  UngainTsProdOutMax=[]  ClampingZeroOutDataTypeStr=Inherit: Inherit via back propagation  ClampingZeroOutMin=[]  ClampingZeroOutMax=[]  FilterDenConstantOutDataTypeStr=Inherit: Inherit via back propagation  FilterDenConstantOutMin=[]  FilterDenConstantOutMax=[]  PCopyOutDataTypeStr=Inherit: Inherit via back propagation  PCopyOutMin=[]  PCopyOutMax=[]  NCopyOutDataTypeStr=Inherit: Inherit via back propagation  NCopyOutMin=[]  NCopyOutMax=[]  IntegratorContinuousStateAttributes=''  IntegratorStateMustResolveToSignalObject=off  IntegratorRTWStateStorageClass=Auto  FilterContinuousStateAttributes=''  FilterStateMustResolveToSignalObject=off  FilterRTWStateStorageClass=Auto  ParallelPVariant=InternalParameters  IdealPVariant=Disabled  IVariant=InternalParameters  DVariant=Disabled  IntegratorVariant=Discrete  SatVariant=Enabled  AWVariant=BackCalculation  PCopyVariant=Disabled  TRVariant=Disabled  FdbkBlocksVariant=Forward  IdealPFdbkVariant=Disabled  SatFdbkVariant=Disabled  DerivativeFilterVariant=Disabled  NVariant=Disabled  NCopyVariant=Disabled_SignalSpec  FilterICVariant=Disabled  IntegratorICVariant=InternalICs  ExternalResetVariant=Disabled  TRSumVariant=Passthrough  SumFdbkVariant=Disabled  SumVariant=Sum_PI  TsampFilterVariant=InternalTs  TsampNgainVariant=Passthrough  TsampIntegralVariant=Disabled_SignalSpec  ExternalSaturationOutDataTypeStr=Inherit: Same as second input  DerivativeSourceVariant=Disabled  PreIntVariant=InternalPreInt
  PI1 : slpidlib/PID Controller  Commented=on  Controller=PI  Form=Parallel  TimeDomain=Discrete-time  UseExternalTs=off  SampleTime=Ts_Control  IntegratorMethod=Forward Euler  FilterMethod=Forward Euler  ControllerParametersSource=internal  P=Kp_Ireg  I=Ki_Ireg  UseKiTs=off  D=0  UseExternalDerivativeSource=off  N=100  UseFilter=on  TunerSelectOption=Transfer Function Based (PID Tuner App)  InitialConditionSource=internal  InitialConditionForIntegrator=0  InitialConditionForFilter=0  DifferentiatorICPrevScaledInput=0  ExternalReset=none  TrackingMode=off  Kt=1  LimitOutput=on  SatLimitsSource=internal  UpperSaturationLimit=1.5  LowerSaturationLimit=-1.5  LinearizeAsGain=off  AntiWindupMode=clamping  Kb=1  LimitIntegrator=off  UpperIntegratorSaturationLimit=inf  LowerIntegratorSaturationLimit=-inf  POutMin=[]  POutMax=[]  IOutMin=[]  IOutMax=[]  DOutMin=[]  DOutMax=[]  NOutMin=[]  NOutMax=[]  SumOutMin=[]  SumOutMax=[]  SaturationOutMin=[]  SaturationOutMax=[]  PParamMin=[]  PParamMax=[]  IParamMin=[]  IParamMax=[]  DParamMin=[]  DParamMax=[]  NParamMin=[]  NParamMax=[]  KbParamMin=[]  KbParamMax=[]  KtParamMin=[]  KtParamMax=[]  KbOutMin=[]  KbOutMax=[]  KtOutMin=[]  KtOutMax=[]  IntegratorOutMin=[]  IntegratorOutMax=[]  FilterOutMin=[]  FilterOutMax=[]  SumI1OutMin=[]  SumI1OutMax=[]  SumI2OutMin=[]  SumI2OutMax=[]  SumI3OutMin=[]  SumI3OutMax=[]  SumI4OutMin=[]  SumI4OutMax=[]  SumDOutMin=[]  SumDOutMax=[]  DifferentiatorOutMin=[]  DifferentiatorOutMax=[]  FilterDiffOutCoefMin=[]  FilterDiffOutCoefMax=[]  ReciprocalOutMin=[]  ReciprocalOutMax=[]  SumDenOutMin=[]  SumDenOutMax=[]  SumNumOutMin=[]  SumNumOutMax=[]  DivideOutMin=[]  DivideOutMax=[]  UdiffTsProdOutMin=[]  UdiffTsProdOutMax=[]  NTsProdOutMin=[]  NTsProdOutMax=[]  UintegralTsProdOutMin=[]  UintegralTsProdOutMax=[]  UngainTsProdOutMin=[]  UngainTsProdOutMax=[]  ClampingZeroOutDataTypeStr=Inherit: Inherit via back propagation  ClampingZeroOutMin=[]  ClampingZeroOutMax=[]  FilterDenConstantOutDataTypeStr=Inherit: Inherit via back propagation  FilterDenConstantOutMin=[]  FilterDenConstantOutMax=[]  PCopyOutDataTypeStr=Inherit: Inherit via back propagation  PCopyOutMin=[]  PCopyOutMax=[]  NCopyOutDataTypeStr=Inherit: Inherit via back propagation  NCopyOutMin=[]  NCopyOutMax=[]  IntegratorContinuousStateAttributes=''  IntegratorStateMustResolveToSignalObject=off  IntegratorRTWStateStorageClass=Auto  FilterContinuousStateAttributes=''  FilterStateMustResolveToSignalObject=off  FilterRTWStateStorageClass=Auto  ParallelPVariant=InternalParameters  IdealPVariant=Disabled  IVariant=InternalParameters  DVariant=Disabled  IntegratorVariant=Discrete  SatVariant=Enabled  AWVariant=DiscClampingParallel  PCopyVariant=Disabled  TRVariant=Disabled  FdbkBlocksVariant=Forward  IdealPFdbkVariant=Disabled  SatFdbkVariant=Disabled  DerivativeFilterVariant=Disabled  NVariant=Disabled  NCopyVariant=Disabled_SignalSpec  FilterICVariant=Disabled  IntegratorICVariant=InternalICs  ExternalResetVariant=Disabled  TRSumVariant=Passthrough  SumFdbkVariant=Disabled  SumVariant=Sum_PI  TsampFilterVariant=InternalTs  TsampNgainVariant=Passthrough  TsampIntegralVariant=Disabled_SignalSpec  ExternalSaturationOutDataTypeStr=Inherit: Same as second input  DerivativeSourceVariant=Disabled  PreIntVariant=InternalPreInt
  PI2 : slpidlib/PID Controller  Commented=on  Controller=PI  Form=Parallel  TimeDomain=Discrete-time  UseExternalTs=off  SampleTime=Ts_Control  IntegratorMethod=Forward Euler  FilterMethod=Forward Euler  ControllerParametersSource=internal  P=Kp_Ireg  I=Ki_Ireg  UseKiTs=off  D=0  UseExternalDerivativeSource=off  N=100  UseFilter=on  TunerSelectOption=Transfer Function Based (PID Tuner App)  InitialConditionSource=internal  InitialConditionForIntegrator=0  InitialConditionForFilter=0  DifferentiatorICPrevScaledInput=0  ExternalReset=none  TrackingMode=off  Kt=1  LimitOutput=on  SatLimitsSource=internal  UpperSaturationLimit=1.5  LowerSaturationLimit=-1.5  LinearizeAsGain=off  AntiWindupMode=back-calculation  Kb=1  LimitIntegrator=off  UpperIntegratorSaturationLimit=inf  LowerIntegratorSaturationLimit=-inf  POutMin=[]  POutMax=[]  IOutMin=[]  IOutMax=[]  DOutMin=[]  DOutMax=[]  NOutMin=[]  NOutMax=[]  SumOutMin=[]  SumOutMax=[]  SaturationOutMin=[]  SaturationOutMax=[]  PParamMin=[]  PParamMax=[]  IParamMin=[]  IParamMax=[]  DParamMin=[]  DParamMax=[]  NParamMin=[]  NParamMax=[]  KbParamMin=[]  KbParamMax=[]  KtParamMin=[]  KtParamMax=[]  KbOutMin=[]  KbOutMax=[]  KtOutMin=[]  KtOutMax=[]  IntegratorOutMin=[]  IntegratorOutMax=[]  FilterOutMin=[]  FilterOutMax=[]  SumI1OutMin=[]  SumI1OutMax=[]  SumI2OutMin=[]  SumI2OutMax=[]  SumI3OutMin=[]  SumI3OutMax=[]  SumI4OutMin=[]  SumI4OutMax=[]  SumDOutMin=[]  SumDOutMax=[]  DifferentiatorOutMin=[]  DifferentiatorOutMax=[]  FilterDiffOutCoefMin=[]  FilterDiffOutCoefMax=[]  ReciprocalOutMin=[]  ReciprocalOutMax=[]  SumDenOutMin=[]  SumDenOutMax=[]  SumNumOutMin=[]  SumNumOutMax=[]  DivideOutMin=[]  DivideOutMax=[]  UdiffTsProdOutMin=[]  UdiffTsProdOutMax=[]  NTsProdOutMin=[]  NTsProdOutMax=[]  UintegralTsProdOutMin=[]  UintegralTsProdOutMax=[]  UngainTsProdOutMin=[]  UngainTsProdOutMax=[]  ClampingZeroOutDataTypeStr=Inherit: Inherit via back propagation  ClampingZeroOutMin=[]  ClampingZeroOutMax=[]  FilterDenConstantOutDataTypeStr=Inherit: Inherit via back propagation  FilterDenConstantOutMin=[]  FilterDenConstantOutMax=[]  PCopyOutDataTypeStr=Inherit: Inherit via back propagation  PCopyOutMin=[]  PCopyOutMax=[]  NCopyOutDataTypeStr=Inherit: Inherit via back propagation  NCopyOutMin=[]  NCopyOutMax=[]  IntegratorContinuousStateAttributes=''  IntegratorStateMustResolveToSignalObject=off  IntegratorRTWStateStorageClass=Auto  FilterContinuousStateAttributes=''  FilterStateMustResolveToSignalObject=off  FilterRTWStateStorageClass=Auto  ParallelPVariant=InternalParameters  IdealPVariant=Disabled  IVariant=InternalParameters  DVariant=Disabled  IntegratorVariant=Discrete  SatVariant=Enabled  AWVariant=BackCalculation  PCopyVariant=Disabled  TRVariant=Disabled  FdbkBlocksVariant=Forward  IdealPFdbkVariant=Disabled  SatFdbkVariant=Disabled  DerivativeFilterVariant=Disabled  NVariant=Disabled  NCopyVariant=Disabled_SignalSpec  FilterICVariant=Disabled  IntegratorICVariant=InternalICs  ExternalResetVariant=Disabled  TRSumVariant=Passthrough  SumFdbkVariant=Disabled  SumVariant=Sum_PI  TsampFilterVariant=InternalTs  TsampNgainVariant=Passthrough  TsampIntegralVariant=Disabled_SignalSpec  ExternalSaturationOutDataTypeStr=Inherit: Same as second input  DerivativeSourceVariant=Disabled  PreIntVariant=InternalPreInt
  Rff : Gain  Commented=on  Gain=inv1.R/inv1.Zb  SaturateOnIntegerOverflow=on  OutDataTypeStr=Inherit: Same as input  ParamDataTypeStr=Inherit: Same as input
  "Rff " : Gain  Commented=on  Gain=inv1.R/inv1.Zb  SaturateOnIntegerOverflow=on  OutDataTypeStr=Inherit: Same as input  ParamDataTypeStr=Inherit: Same as input
  Rff 1 : Gain  Commented=on  Gain=Rtot_pu  SaturateOnIntegerOverflow=on  OutDataTypeStr=Inherit: Same as input  ParamDataTypeStr=Inherit: Same as input
  Saturation : Saturate  UpperLimit=1.5  LowerLimit=-1.5
  Scope : Scope  NumInputPorts=2
  Scope1 : Scope
  Sum : Sum  Inputs=|-+
  VdVq_conv : Outport  VectorParamsAs1DForOutWhenUnconnected=off
  wires:
  Mux/1 -> Add2/2
  PI/1 -> Scope/2, Add2/1  "PI"
  Sum/1 -> Scope/1, PI/1
  IdIq_ref/1 -> Sum/2
  IdIq_meas/1 -> Demux1/1, Sum/1
  Add2/1 -> Saturation/1
  Saturation/1 -> Scope1/1, VdVq_conv/1
  VdVq_meas/1 -> Demux/1
  Demux/1 -> Add1/1
  "Rff "/1 -> Add1/2
  Demux1/1 -> "Rff "/1, Lff/1
  "Lff  "/1 -> Add1/3
  Demux1/2 -> "Lff  "/1, Rff/1
  Rff/1 -> Add3/2
  Lff/1 -> Add3/3
  Add1/1 -> Mux/1  "Feedforward"
  Demux/2 -> Add3/1
  Add3/1 -> Mux/2

== system different_inverter_controls_BPS/IBR-GFM PV Droop/IBR/Inverter Control/Current Control/Uabc_ref Generation max (m) = 1 ==
  note: (Correction for transformer
      |  D1 connection)
  note: (Correction for delay of Ts_Control)
  note: Uref Generation
      | ==============
  wt : Inport
  VdVq_conv : Inport  Port=2
  Add1 : Sum  Inputs=++++
  Add2 : Sum
  Complex to Magnitude-Angle : ComplexToMagnitudeAngle
  Constant : Constant  Commented=on  Value=-pi/6
  Constant1 : Constant  Commented=on  Value=Vnom_dc
  Constant2 : Constant  Value="[ 0  -2*pi/3  2*pi/3  ]"
  Constant3 : Constant  Commented=on  Value=Vnom_sec*sqrt(2)/sqrt(3)
  Constant4 : Constant  Value=Ts_Control*Fnom*(2*pi)
  Constant5 : Constant  Value=Vdc
  Constant6 : Constant  Value=Vpp*sqrt(2)/sqrt(3)
  Demux1 : Demux  Outputs=2
  Gain1 : Gain  Gain=1/2
  Product : Product  Inputs=*/  RndMeth=Zero
  Product1 : Product  Inputs=*/  RndMeth=Zero
  Product2 : Product  Inputs=**  RndMeth=Zero
  Real-Imag to Complex : RealImagToComplex
  Trigonometric Function : Trigonometry
  Uabc_ref : Outport  VectorParamsAs1DForOutWhenUnconnected=off
  wires:
  Constant5/1 -> Gain1/1
  VdVq_conv/1 -> Product1/1
  Product1/1 -> Demux1/1
  Gain1/1 -> Product/1
  Real-Imag to Complex/1 -> Complex to Magnitude-Angle/1
  Demux1/1 -> Real-Imag to Complex/1
  Demux1/2 -> Real-Imag to Complex/2
  Constant2/1 -> Add1/2
  Constant/1 -> Add1/3
  Constant6/1 -> Product/2
  Complex to Magnitude-Angle/2 -> Add2/1
  Add1/1 -> Add2/2
  Add2/1 -> Trigonometric Function/1
  Complex to Magnitude-Angle/1 -> Product2/1
  Trigonometric Function/1 -> Product2/2
  Product2/1 -> Uabc_ref/1
  wt/1 -> Add1/1
  Constant4/1 -> Add1/4
  Product/1 -> Product1/2

== system different_inverter_controls_BPS/IBR-GFM PV Droop/IBR/Inverter Control/current limiter/P priority limit ==
  idiqP : Inport
  Demux4 : Demux  Outputs=2
  IqLimit : Subsystem
  Mux4 : Mux  Inputs=2
  Rtot_pu1 : Gain  Gain=-1  SaturateOnIntegerOverflow=on  OutDataTypeStr=Inherit: Same as input  ParamDataTypeStr=Inherit: Same as input
  Saturation : Saturate  UpperLimit=limMax  LowerLimit=0
  Saturation Dynamic : simulink/Discontinuities/Saturation Dynamic  OutMin=[]  OutMax=[limMax]  OutDataTypeStr=Inherit: Same as second input  OutDataType=fixdt(1, 16)  OutScaling=2^-10  DoSatur=off
  idiqPRefL : Outport
  wires:
  IqLimit/1(Out2) -> Saturation Dynamic/1, Rtot_pu1/1
  Rtot_pu1/1 -> Saturation Dynamic/3
  Saturation/1 -> Mux4/1, IqLimit/1(In1)
  Demux4/1 -> Saturation/1
  Mux4/1 -> idiqPRefL/1
  Demux4/2 -> Saturation Dynamic/2
  idiqP/1 -> Demux4/1
  Saturation Dynamic/1 -> Mux4/2

== system different_inverter_controls_BPS/IBR-GFM PV Droop/IBR/Inverter Control/current limiter/Q priority limit ==
  idiqP : Inport
  V_inv_mag : Inport  Port=2
  Demux4 : Demux  Outputs=2
  Iq condition : Switch  Threshold=0.9  SaturateOnIntegerOverflow=off  InputSameDT=off
  IqLimit : Subsystem
  Mux4 : Mux  Inputs=2
  Rtot_pu1 : Gain  Gain=-1  SaturateOnIntegerOverflow=on  OutDataTypeStr=Inherit: Same as input  ParamDataTypeStr=Inherit: Same as input
  Saturation : Saturate  UpperLimit=limMax  LowerLimit=limMin
  Saturation Dynamic : simulink/Discontinuities/Saturation Dynamic  OutMin=[]  OutMax=[]  OutDataTypeStr=Inherit: Same as second input  OutDataType=fixdt(1, 16)  OutScaling=2^-10  DoSatur=off
  Saturation1 : Saturate  UpperLimit=0  LowerLimit=limMin
  Scope : Scope
  idiqPRefL : Outport
  wires:
  Demux4/2 -> Saturation1/1, Saturation/1
  Saturation1/1 -> Iq condition/3
  IqLimit/1(Out2) -> Saturation Dynamic/1, Rtot_pu1/1
  Demux4/1 -> Saturation Dynamic/2
  Saturation Dynamic/1 -> Mux4/1
  Rtot_pu1/1 -> Saturation Dynamic/3
  Mux4/1 -> idiqPRefL/1
  idiqP/1 -> Demux4/1
  Saturation/1 -> Iq condition/1
  V_inv_mag/1 -> Iq condition/2
  Iq condition/1 -> IqLimit/1(In1), Mux4/2

== system different_inverter_controls_BPS/IBR-GFM PV Droop/IBR/Inverter Control/current limiter/Subsystem3 ==
  In1 : Inport
  Demux2 : Demux  Outputs=2
  Math Function : Math  Operator=square  SignedPower=on
  Saturation : Saturate  UpperLimit=limMax  LowerLimit=limMin
  Scope : Scope  NumInputPorts=2
  Sqrt1 : Sqrt
  Subtract : Sum
  Out1 : Outport
  Out2 : Outport  Port=2
  wires:
  Saturation/1 -> Out1/1
  Sqrt1/1 -> Out2/1, Scope/1, Saturation/1
  Subtract/1 -> Sqrt1/1  "Ipos2"
  In1/1 -> Math Function/1, Scope/2
  Math Function/1 -> Demux2/1
  Demux2/1 -> Subtract/1
  Demux2/2 -> Subtract/2

== system different_inverter_controls_BPS/IBR-GFM PV Droop/IBR/Inverter Control/current limiter/Subsystem4 ==
  In1 : Inport
  In2 : Inport  Port=2
  Demux4 : Demux  Outputs=2
  Mux4 : Mux  Inputs=2
  Switch1 : Switch  Threshold=limMax  SaturateOnIntegerOverflow=off  InputSameDT=off
  Unit Delay2 : UnitDelay  InitialCondition=1  SampleTime=Ts_Control  HasFrameUpgradeWarning=on
  dummy limit : Saturate  UpperLimit=limMax  LowerLimit=limMin
  Out1 : Outport
  wires:
  dummy limit/1 -> Mux4/2
  Demux4/2 -> dummy limit/1
  In2/1 -> Demux4/1, Switch1/3
  In1/1 -> Switch1/2
  Unit Delay2/1 -> Switch1/1
  Switch1/1 -> Unit Delay2/1, Mux4/1, Out1/1

== system different_inverter_controls_BPS/IBR-GFM PV Droop/IBR/Inverter Control/current limiter/Subsystem9 ==
  In1 : Inport
  In2 : Inport  Port=2
  Divide : Product  Inputs=*/
  Gain1 : Gain  Gain=limMax
  Saturation : Saturate  UpperLimit=limMax  LowerLimit=limMin
  Switch1 : Switch  Threshold=limMax  SaturateOnIntegerOverflow=off  InputSameDT=off
  idiqPRefL : Outport
  wires:
  Saturation/1 -> idiqPRefL/1
  Switch1/1 -> Saturation/1
  Gain1/1 -> Switch1/1
  Divide/1 -> Gain1/1
  In2/1 -> Switch1/3, Divide/1
  In1/1 -> Switch1/2, Divide/2

== system different_inverter_controls_BPS/IBR-GFM PV Droop/IBR/Power Controller/P,Q Control /Integrator ==
  w : Inport
  Constant1 : Constant  Commented=on  Value=2*pi  SampleTime=Ts
  Constant2 : Constant  Value=2*pi  SampleTime=Ts_Control
  Constant3 : Constant  Commented=on  Value=2*pi  SampleTime=Ts
  Constant4 : Constant  Commented=on  Value=f  SampleTime=Ts_Control
  Constant5 : Constant  Commented=on  Value=0  SampleTime=Ts_Control
  Discrete-Time Integrator : DiscreteIntegrator  Commented=on  IntegratorMethod=Integration: Trapezoidal  SampleTime=Ts  ICPrevOutput=DiscIntNeverNeededParam  ICPrevScaledInput=DiscIntNeverNeededParam
  Discrete-Time Integrator1 : DiscreteIntegrator  ExternalReset=rising  InitialConditionSource=external  SampleTime=Ts_Control  ShowStatePort=on  ICPrevOutput=DiscIntNeverNeededParam  ICPrevScaledInput=DiscIntNeverNeededParam
  Divide : Product  Commented=on  Inputs=*/
  From : From  Commented=on  GotoTag=fsys
  Gain : Gain  Commented=on  Gain=2*pi*f
  Gain1 : Gain  Commented=on  Gain=2*pi*f  SaturateOnIntegerOverflow=on  OutDataTypeStr=Inherit: Same as input  ParamDataTypeStr=Inherit: Same as input
  Gain3 : Gain  Gain=2*pi*f
  Hit Crossing : HitCross  Commented=on  HitCrossingOffset=pi  HitCrossingDirection=falling  ShowOutputPort=off
  Initial : InitialCondition  Value=0
  Initial1 : InitialCondition  Commented=on  Value=0
  Integrator : Integrator  Commented=on  ExternalReset=rising  InitialConditionSource=external  InitialCondition=sps.Phase_Init*pi/180  LimitOutput=on  ShowStatePort=on
  Integrator2 : Integrator  Commented=on  ExternalReset=rising  InitialConditionSource=external  InitialCondition=sps.Phase_Init*pi/180  ShowStatePort=on
  Math Function : Math  Commented=on  Operator=mod  SignedPower=on
  Relational Operator : RelationalOperator  Operator=>  OutDataTypeStr=boolean  InputSameDT=off
  Relational Operator1 : RelationalOperator  Commented=on  Operator=>  OutDataTypeStr=boolean  InputSameDT=off
  Scope : Scope
  Scope1 : Scope  Commented=on
  Scope2 : Scope  Commented=on
  Scope3 : Scope  Commented=on
  Subtract : Sum  Inputs=+-
  Subtract1 : Sum  Commented=on  Inputs=+-
  Sum1 : Sum  Commented=on  Inputs=|++
  Sum2 : Sum  Commented=on  Inputs=|+-
  Theta : Outport
  wires:
  Divide/1 -> Sum1/2
  Constant4/1 -> Divide/2
  From/1 -> Divide/1
  Sum2/1 -> Sum1/1, Scope2/1  "W"
  Constant5/1 -> Sum2/2
  Sum1/1 -> Gain/1  "W"
  Math Function/1 -> Scope1/1
  Constant3/1 -> Math Function/2
  Discrete-Time Integrator/1 -> Math Function/1
  Gain/1 -> Discrete-Time Integrator/1
  Discrete-Time Integrator1/1 -> Theta/1, Scope/1
  Subtract/1 -> Initial/1
  Constant2/1 -> Relational Operator/2, Subtract/2
  Discrete-Time Integrator1/State -> Relational Operator/1, Subtract/1
  Initial/1 -> Discrete-Time Integrator1/3
  Relational Operator/1 -> Discrete-Time Integrator1/2
  Subtract1/1 -> Initial1/1
  Integrator/1 -> Hit Crossing/1, Scope3/1
  Constant1/1 -> Relational Operator1/2, Subtract1/2
  Integrator/State -> Relational Operator1/1, Subtract1/1
  Relational Operator1/1 -> Integrator/2
  Initial1/1 -> Integrator/3
  Gain1/1 -> Integrator/1
  w/1 -> Gain3/1, Sum2/1
  Gain3/1 -> Discrete-Time Integrator1/1
